simulink model "motor_pid_model"  (R2018a)
settings: Solver=VariableStepAuto  StartTime=0.0  StopTime=1  FixedStep=1e-4  RelTol=1e-3
InitFcn:
  | Tw=0.02;     %Ancho de Ventana
  | ppv=20;      %Pulsos por vuelta
  | Ts=1e-4;     %Tiempo de muestreo
  | 
  | Kp=0.002;
  | Kd=0.0009;
  | Ki=20;
  | N=100;
  | h=0.02;
  | 
  | % Los valores de num, den se obtienen de punto_2.m
  | % Fueron hardcodeados por comodidad.
  | 
  | num = [0 0.7770 0];
  | den = [1.0000 -0.9918 -0.006138];
settings Model: Creator=Martin  LastModifiedBy=Alan
settings CodeAppCC: StateflowObjectComments=on

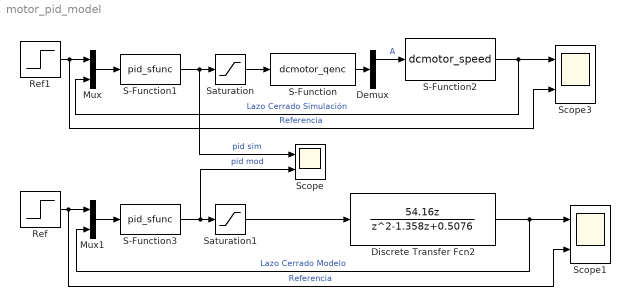
== system motor_pid_model ==
  Demux : Demux  Outputs=2
  Discrete Transfer Fcn2 : DiscreteTransferFcn  Numerator=[54.16 0]  Denominator=[1 -1.358 +0.5076]  SampleTime=Tw
  Mux : Mux  Inputs=2
  Mux1 : Mux  Inputs=2
  Ref : Step  Time=0.2  After=4200  SampleTime=0
  Ref1 : Step  Time=0.2  After=4200  SampleTime=0
  S-Function : S-Function  FunctionName=dcmotor_qenc  Parameters=ppv  SFunctionDeploymentMode=off  EnableBusSupport=off
  S-Function1 : S-Function  FunctionName=pid_sfunc  Parameters=Kp,Kd,Ki,N,h  SFunctionDeploymentMode=off  EnableBusSupport=off
  S-Function2 : S-Function  FunctionName=dcmotor_speed  Parameters=Ts,ppv,Tw  SFunctionDeploymentMode=off  EnableBusSupport=off
  S-Function3 : S-Function  FunctionName=pid_sfunc  Parameters=Kp,Kd,Ki,N,h  SFunctionDeploymentMode=off  EnableBusSupport=off
  Saturation : Saturate  UpperLimit=30  LowerLimit=-30
  Saturation1 : Saturate  UpperLimit=30  LowerLimit=-30
  Scope : Scope  NumInputPorts=2
  Scope1 : Scope  NumInputPorts=2
  Scope3 : Scope  NumInputPorts=2
  wires:
  Ref/1 -> Scope1/2, Mux1/1  "Referencia"
  S-Function/1 -> Demux/1
  Demux/1 -> S-Function2/1  "A"
  S-Function2/1 -> Scope3/1, Mux/2  "Lazo Cerrado Simulación"
  Mux/1 -> S-Function1/1
  Saturation/1 -> S-Function/1
  S-Function1/1 -> Saturation/1, Scope/1  "pid sim"
  Mux1/1 -> S-Function3/1
  S-Function3/1 -> Scope/2, Saturation1/1  "pid mod"
  Saturation1/1 -> Discrete Transfer Fcn2/1
  Discrete Transfer Fcn2/1 -> Mux1/2, Scope1/1  "Lazo Cerrado Modelo"
  Ref1/1 -> Mux/1, Scope3/2  "Referencia"
